simulink model "adelanto_final"  (Simulink 7.5)
settings: Solver=ode45  StartTime=1.8  StopTime=4.5  FixedStep=1/10  RelTol=1e-3
libraries: fl_lib x56, nesl_utility x6, simulink x1
settings Model: Creator=davito  LastModifiedBy=davito
settings SFSimCC: SimCustomSourceCode=|
  | shh = get(0,'ShowHiddenHandles');
  | set(0,'ShowHiddenHandles','On')
  | set(gcf,'menubar','figure')
  | set(gcf,'CloseRequestFcn','closereq')
  | set(gcf,'DefaultLineClipping','Off')
  | set(0,'ShowHiddenHandles',shh)

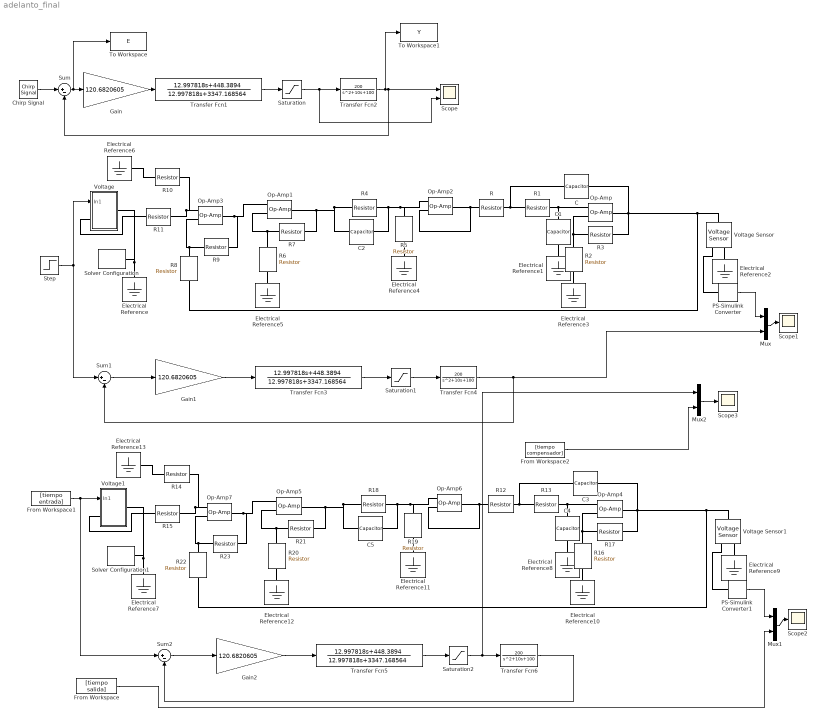
== system adelanto_final ==
  C{,1..5} (6 alike) : fl_lib/Electrical/Electrical Elements/Capacitor  DialogController=NetworkEngine.DynNeDlgSource  SystemSampleTime=-1  c=10e-6 F  v0=0 V  r=1e-6 Ohm  g=0 1/Ohm  i_Log=off  v_Log=off  vc_Log=off  LocalVarNames=|i|v|vc  LocalVarDescs=|i|v|Internal variable for voltage across capacitor term  LocalVarLogging=[0 0 0]
  Chirp Signal : simulink/Sources/Chirp Signal  SystemSampleTime=-1  f1=0.1  T=200  f2=30
  Electrical Reference{,1..13} (14 alike) : fl_lib/Electrical/Electrical Elements/Electrical Reference  DialogController=NetworkEngine.DynNeDlgSource  SystemSampleTime=-1  i_Log=off  LocalVarNames=|i  LocalVarDescs=|i  LocalVarLogging=0
  From Workspace : FromWorkspace  VariableName=[tiempo salida]  SampleTime=0.019959250000000
  From Workspace1 : FromWorkspace  VariableName=[tiempo entrada]  SampleTime=0.019959250000000
  From Workspace2 : FromWorkspace  VariableName=[tiempo compensador]  SampleTime=0.019959250000000
  Gain : Gain  Gain=120.6820605  ParameterDataType=fixdt(1, 16)  ParameterScaling=2^0  OutDataType=fixdt(1, 16)  OutScaling=2^0
  Gain1 : Gain  Gain=120.6820605  ParameterDataType=fixdt(1, 16)  ParameterScaling=2^0  OutDataType=fixdt(1, 16)  OutScaling=2^0
  Gain2 : Gain  Gain=120.6820605  ParameterDataType=fixdt(1, 16)  ParameterScaling=2^0  OutDataType=fixdt(1, 16)  OutScaling=2^0
  Mux : Mux  Inputs=2
  Mux1 : Mux  Inputs=2
  Mux2 : Mux  Inputs=2
  Op-Amp{,1..7} (8 alike) : fl_lib/Electrical/Electrical Elements/Op-Amp  DialogController=NetworkEngine.DynNeDlgSource  SystemSampleTime=-1  i1_Log=off  v1_Log=off  outI_Log=off  LocalVarNames=|i1|v1|outI  LocalVarDescs=|i1|v1|outI  LocalVarLogging=[0 0 0]
  PS-Simulink Converter : nesl_utility/PS-Simulink Converter  DialogController=NetworkEngine.DynNeUtilDlgSource  SystemSampleTime=-1  PhysicalDomain=network_engine_domain  LeftPortType=input  RightPortType=output  SubClassName=ps_output  Unit=1  AffineConversion=off
  PS-Simulink Converter1 : nesl_utility/PS-Simulink Converter  DialogController=NetworkEngine.DynNeUtilDlgSource  SystemSampleTime=-1  PhysicalDomain=network_engine_domain  LeftPortType=input  RightPortType=output  SubClassName=ps_output  Unit=1  AffineConversion=off
  R{,1,12..13} (4 alike) : fl_lib/Electrical/Electrical Elements/Resistor  DialogController=NetworkEngine.DynNeDlgSource  SystemSampleTime=-1  R=10 kOhm  i_Log=off  v_Log=off  LocalVarNames=|i|v  LocalVarDescs=|i|v  LocalVarLogging=[0 0]
  R{8..11,14..15,22..23} (8 alike) : fl_lib/Electrical/Electrical Elements/Resistor  DialogController=NetworkEngine.DynNeDlgSource  SystemSampleTime=-1  R=1 kOhm  i_Log=off  v_Log=off  LocalVarNames=|i|v  LocalVarDescs=|i|v  LocalVarLogging=[0 0]
  R{2..3,16..17} (4 alike) : fl_lib/Electrical/Electrical Elements/Resistor  DialogController=NetworkEngine.DynNeDlgSource  SystemSampleTime=-1  R=4.7 kOhm  i_Log=off  v_Log=off  LocalVarNames=|i|v  LocalVarDescs=|i|v  LocalVarLogging=[0 0]
  R18 : fl_lib/Electrical/Electrical Elements/Resistor  DialogController=NetworkEngine.DynNeDlgSource  SystemSampleTime=-1  R=2.898779149 kOhm  i_Log=off  v_Log=off  LocalVarNames=|i|v  LocalVarDescs=|i|v  LocalVarLogging=[0 0]
  R19 : fl_lib/Electrical/Electrical Elements/Resistor  DialogController=NetworkEngine.DynNeDlgSource  SystemSampleTime=-1  R=448.3894145 Ohm  i_Log=off  v_Log=off  LocalVarNames=|i|v  LocalVarDescs=|i|v  LocalVarLogging=[0 0]
  R20 : fl_lib/Electrical/Electrical Elements/Resistor  DialogController=NetworkEngine.DynNeDlgSource  SystemSampleTime=-1  R=2 kOhm  i_Log=off  v_Log=off  LocalVarNames=|i|v  LocalVarDescs=|i|v  LocalVarLogging=[0 0]
  R21 : fl_lib/Electrical/Electrical Elements/Resistor  DialogController=NetworkEngine.DynNeDlgSource  SystemSampleTime=-1  R=239.3618 kOhm  i_Log=off  v_Log=off  LocalVarNames=|i|v  LocalVarDescs=|i|v  LocalVarLogging=[0 0]
  R4 : fl_lib/Electrical/Electrical Elements/Resistor  DialogController=NetworkEngine.DynNeDlgSource  SystemSampleTime=-1  R=2.898779149 kOhm  i_Log=off  v_Log=off  LocalVarNames=|i|v  LocalVarDescs=|i|v  LocalVarLogging=[0 0]
  R5 : fl_lib/Electrical/Electrical Elements/Resistor  DialogController=NetworkEngine.DynNeDlgSource  SystemSampleTime=-1  R=448.3894145 Ohm  i_Log=off  v_Log=off  LocalVarNames=|i|v  LocalVarDescs=|i|v  LocalVarLogging=[0 0]
  R6 : fl_lib/Electrical/Electrical Elements/Resistor  DialogController=NetworkEngine.DynNeDlgSource  SystemSampleTime=-1  R=2 kOhm  i_Log=off  v_Log=off  LocalVarNames=|i|v  LocalVarDescs=|i|v  LocalVarLogging=[0 0]
  R7 : fl_lib/Electrical/Electrical Elements/Resistor  DialogController=NetworkEngine.DynNeDlgSource  SystemSampleTime=-1  R=239.3618 kOhm  i_Log=off  v_Log=off  LocalVarNames=|i|v  LocalVarDescs=|i|v  LocalVarLogging=[0 0]
  Saturation : Saturate  UpperLimit=11  LowerLimit=-11  OutDataType=fixdt(1, 16)  OutScaling=2^0
  Saturation1 : Saturate  UpperLimit=11  LowerLimit=-11  OutDataType=fixdt(1, 16)  OutScaling=2^0
  Saturation2 : Saturate  UpperLimit=11  LowerLimit=-11  OutDataType=fixdt(1, 16)  OutScaling=2^0
  Scope : Scope  NumInputPorts=2
      settings: YMin=-5~-5  YMax=5~5
  Scope1 : Scope
      settings: YMin=0.93  YMax=1.06
  Scope2 : Scope
      settings: YMin=0  YMax=1.05e-20  SaveName=ScopeData2
  Scope3 : Scope
      settings: YMin=0  YMax=1.05e-20  SaveName=ScopeData3
  Solver Configuration : nesl_utility/Solver Configuration  DialogController=NetworkEngine.DynNeUtilDlgSource  SystemSampleTime=-1  PhysicalDomain=network_engine_domain  LeftPortType=input  RightPortType=generic  SubClassName=solver  Accelerate=off  Profile=off  ResidualTolerance=1e-9  MaxNonlinIter=3  MaxModeIter=2  DoFixedCost=off  UseLocalSampling=off  DoDC=off  LinearAlgebra=Sparse  LocalSolverSampleTime=.001  LocalSolverChoice=NE_BACKWARD_EULER_ADVANCER  UseLocalSolver=off
  Solver Configuration1 : nesl_utility/Solver Configuration  DialogController=NetworkEngine.DynNeUtilDlgSource  SystemSampleTime=-1  PhysicalDomain=network_engine_domain  LeftPortType=input  RightPortType=generic  SubClassName=solver  Accelerate=off  Profile=off  ResidualTolerance=1e-9  MaxNonlinIter=3  MaxModeIter=2  DoFixedCost=off  UseLocalSampling=off  DoDC=off  LinearAlgebra=Sparse  LocalSolverSampleTime=.001  LocalSolverChoice=NE_BACKWARD_EULER_ADVANCER  UseLocalSolver=off
  Step : Step  Time=0  SampleTime=0
  Sum : Sum  Inputs=|+-  OutDataType=fixdt(1, 16)  OutScaling=2^0
  Sum1 : Sum  Inputs=|+-  OutDataType=fixdt(1, 16)  OutScaling=2^0
  Sum2 : Sum  Inputs=|+-  OutDataType=fixdt(1, 16)  OutScaling=2^0
  To Workspace : ToWorkspace  VariableName=E  SampleTime=-1  SaveFormat=Array
  To Workspace1 : ToWorkspace  VariableName=Y  SampleTime=-1  SaveFormat=Array
  Transfer Fcn1 : TransferFcn  Numerator=[12.997818 448.3894]  Denominator=[12.997818 3347.168564]
  Transfer Fcn2 : TransferFcn  Numerator=[200]  Denominator=[1 10 100]
  Transfer Fcn3 : TransferFcn  Numerator=[12.997818 448.3894]  Denominator=[12.997818 3347.168564]
  Transfer Fcn4 : TransferFcn  Numerator=[200]  Denominator=[1 10 100]
  Transfer Fcn5 : TransferFcn  Numerator=[12.997818 448.3894]  Denominator=[12.997818 3347.168564]
  Transfer Fcn6 : TransferFcn  Numerator=[200]  Denominator=[1 10 100]
  Voltage : Subsystem
  Voltage Sensor : fl_lib/Electrical/Electrical Sensors/Voltage Sensor  DialogController=NetworkEngine.DynNeDlgSource  SystemSampleTime=-1  i1_Log=off  v1_Log=off  LocalVarNames=|i1|v1  LocalVarDescs=|i1|v1  LocalVarLogging=[0 0]
  Voltage Sensor1 : fl_lib/Electrical/Electrical Sensors/Voltage Sensor  DialogController=NetworkEngine.DynNeDlgSource  SystemSampleTime=-1  i1_Log=off  v1_Log=off  LocalVarNames=|i1|v1  LocalVarDescs=|i1|v1  LocalVarLogging=[0 0]
  Voltage1 : Subsystem
  wires:
  Sum/1 -> Gain/1, To Workspace/1
  Gain/1 -> Transfer Fcn1/1
  Transfer Fcn1/1 -> Saturation/1
  Transfer Fcn2/1 -> Sum/2, Scope/1, To Workspace1/1
  Chirp Signal/1 -> Sum/1
  Saturation/1 -> Transfer Fcn2/1, Scope/2
  Step/1 -> Voltage/1(In1), Sum1/1
  PS-Simulink Converter/1 -> Mux/1
  Mux/1 -> Scope1/1
  Gain1/1 -> Transfer Fcn3/1
  Transfer Fcn3/1 -> Saturation1/1
  Transfer Fcn4/1 -> Mux/2, Sum1/2
  Sum1/1 -> Gain1/1
  Saturation1/1 -> Transfer Fcn4/1
  PS-Simulink Converter1/1 -> Mux1/1
  Mux1/1 -> Scope2/1
  Gain2/1 -> Transfer Fcn5/1
  Transfer Fcn5/1 -> Saturation2/1
  Transfer Fcn6/1 -> Sum2/2
  Sum2/1 -> Gain2/1
  Saturation2/1 -> Transfer Fcn6/1, Mux2/1
  From Workspace1/1 -> Voltage1/1(In1), Sum2/1
  Mux2/1 -> Scope3/1
  From Workspace2/1 -> Mux2/2
  From Workspace/1 -> Mux1/2
  connections:
  Voltage/RConn1 -- Solver Configuration/RConn1 -- Electrical Reference/LConn1
  C/LConn1 -- R/RConn1 -- R1/LConn1
  C1/LConn1 -- Op-Amp/LConn1 -- R1/RConn1
  R3/LConn1 -- R2/LConn1 -- Op-Amp/LConn2
  C/RConn1 -- Op-Amp/RConn1 -- R3/RConn1 -- Voltage Sensor/LConn1 -- R8/RConn1
  Voltage Sensor/RConn1 -- PS-Simulink Converter/LConn1
  R2/RConn1 -- Electrical Reference3/LConn1
  Electrical Reference1/LConn1 -- C1/RConn1
  Voltage Sensor/RConn2 -- Electrical Reference2/LConn1
  Op-Amp2/LConn1 -- R4/RConn1 -- C2/LConn1 -- R5/LConn1
  R7/LConn1 -- Op-Amp1/RConn1 -- C2/RConn1 -- R4/LConn1
  R5/RConn1 -- Electrical Reference4/LConn1
  R7/RConn1 -- R6/LConn1 -- Op-Amp1/LConn2
  R6/RConn1 -- Electrical Reference5/LConn1
  Op-Amp2/RConn1 -- R/LConn1 -- Op-Amp2/LConn2
  Op-Amp3/RConn1 -- R9/LConn1 -- Op-Amp1/LConn1
  R9/RConn1 -- Op-Amp3/LConn2 -- R8/LConn1
  R11/LConn1 -- Op-Amp3/LConn1 -- R10/LConn1
  Electrical Reference6/LConn1 -- R10/RConn1
  R11/RConn1 -- Voltage/LConn1
  Voltage1/RConn1 -- Electrical Reference7/LConn1 -- Solver Configuration1/RConn1
  C3/LConn1 -- R13/LConn1 -- R12/RConn1
  Op-Amp4/LConn1 -- C4/LConn1 -- R13/RConn1
  Op-Amp4/LConn2 -- R17/LConn1 -- R16/LConn1
  R22/RConn1 -- Voltage Sensor1/LConn1 -- C3/RConn1 -- R17/RConn1 -- Op-Amp4/RConn1
  Op-Amp6/LConn1 -- R19/LConn1 -- C5/LConn1 -- R18/RConn1
  C5/RConn1 -- R18/LConn1 -- Op-Amp5/RConn1 -- R21/LConn1
  R21/RConn1 -- Op-Amp5/LConn2 -- R20/LConn1
  Op-Amp6/RConn1 -- Op-Amp6/LConn2 -- R12/LConn1
  Op-Amp7/RConn1 -- Op-Amp5/LConn1 -- R23/LConn1
  R23/RConn1 -- R22/LConn1 -- Op-Amp7/LConn2
  R15/LConn1 -- R14/LConn1 -- Op-Amp7/LConn1
  R15/RConn1 -- Voltage1/LConn1
  Electrical Reference13/LConn1 -- R14/RConn1
  R20/RConn1 -- Electrical Reference12/LConn1
  R19/RConn1 -- Electrical Reference11/LConn1
  Voltage Sensor1/RConn2 -- Electrical Reference9/LConn1
  Electrical Reference8/LConn1 -- C4/RConn1
  R16/RConn1 -- Electrical Reference10/LConn1
  Voltage Sensor1/RConn1 -- PS-Simulink Converter1/LConn1

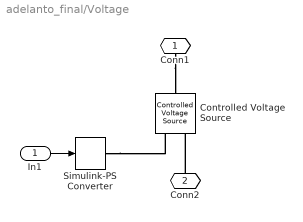
== system adelanto_final/Voltage ==
  In1 : Inport
  Controlled Voltage Source : fl_lib/Electrical/Electrical Sources/Controlled Voltage Source  DialogController=NetworkEngine.DynNeDlgSource  SystemSampleTime=-1  i_Log=off  v_Log=off  LocalVarNames=|i|v  LocalVarDescs=|i|v  LocalVarLogging=[0 0]
  Simulink-PS Converter : nesl_utility/Simulink-PS Converter  DialogController=NetworkEngine.DynNeUtilDlgSource  SystemSampleTime=-1  PhysicalDomain=network_engine_domain  LeftPortType=input  RightPortType=output  SubClassName=ps_input  Unit=1  AffineConversion=off  InputFilterTimeConstant=.001  UdotUserProvided=0
  Conn1 : PMIOPort  Port=1  Side=Left
  Conn2 : PMIOPort  Port=2  Side=Right
  wires:
  In1/1 -> Simulink-PS Converter/1
  connections:
  Simulink-PS Converter/RConn1 -- Controlled Voltage Source/RConn1
  Conn1/RConn1 -- Controlled Voltage Source/LConn1
  Conn2/RConn1 -- Controlled Voltage Source/RConn2

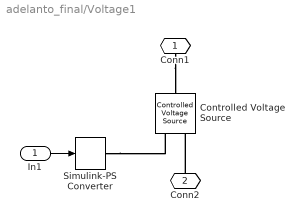
== system adelanto_final/Voltage1 ==
  In1 : Inport
  Controlled Voltage Source : fl_lib/Electrical/Electrical Sources/Controlled Voltage Source  DialogController=NetworkEngine.DynNeDlgSource  SystemSampleTime=-1  i_Log=off  v_Log=off  LocalVarNames=|i|v  LocalVarDescs=|i|v  LocalVarLogging=[0 0]
  Simulink-PS Converter : nesl_utility/Simulink-PS Converter  DialogController=NetworkEngine.DynNeUtilDlgSource  SystemSampleTime=-1  PhysicalDomain=network_engine_domain  LeftPortType=input  RightPortType=output  SubClassName=ps_input  Unit=1  AffineConversion=off  InputFilterTimeConstant=.001  UdotUserProvided=0
  Conn1 : PMIOPort  Port=1  Side=Left
  Conn2 : PMIOPort  Port=2  Side=Right
  wires:
  In1/1 -> Simulink-PS Converter/1
  connections:
  Conn2/RConn1 -- Controlled Voltage Source/RConn2
  Conn1/RConn1 -- Controlled Voltage Source/LConn1
  Simulink-PS Converter/RConn1 -- Controlled Voltage Source/RConn1
